simulink model "Project_3"  (R2020a)
settings: Solver=VariableStepAuto  StartTime=0.0  StopTime=10.0  RelTol=1e-3
settings Model: Creator=hp  LastModifiedBy=hp

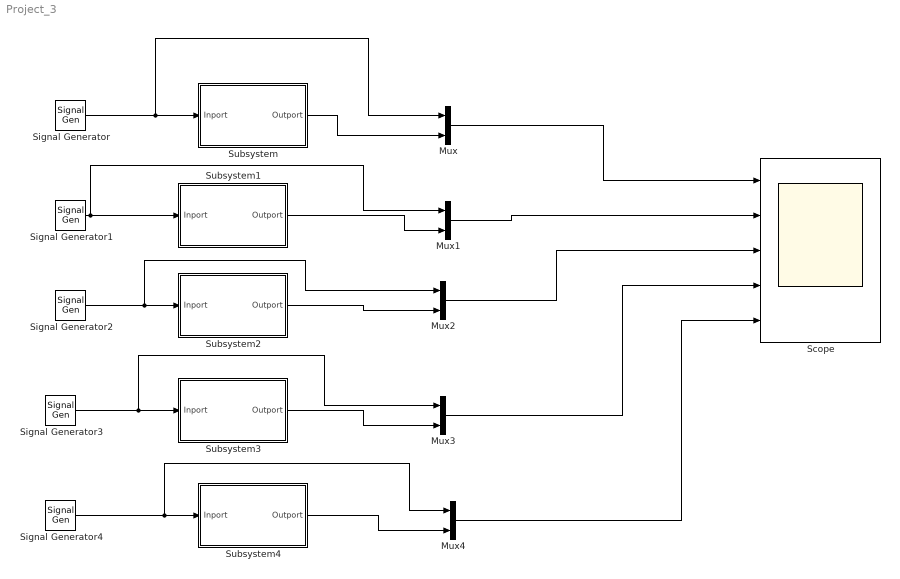
== system Project_3 ==
  Mux{,1..4} (5 alike) : Mux  Inputs=2
  Scope : Scope  NumInputPorts=5
  Signal Generator : SignalGenerator  Frequency=100
  Signal Generator1 : SignalGenerator  Frequency=200  Units=rad/sec
  Signal Generator2 : SignalGenerator  Frequency=500
  Signal Generator3 : SignalGenerator  Frequency=700
  Signal Generator4 : SignalGenerator  Frequency=1000
  Subsystem : Subsystem
  Subsystem1 : Subsystem
  Subsystem2 : Subsystem
  Subsystem3 : Subsystem
  Subsystem4 : Subsystem
  wires:
  Signal Generator4/1 -> Mux4/1, Subsystem4/1(Inport)
  Signal Generator3/1 -> Mux3/1, Subsystem3/1(Inport)
  Signal Generator2/1 -> Mux2/1, Subsystem2/1(Inport)
  Signal Generator/1 -> Mux/1, Subsystem/1(Inport)
  Subsystem/1(Outport) -> Mux/2
  Signal Generator1/1 -> Mux1/1, Subsystem1/1(Inport)
  Subsystem1/1(Outport) -> Mux1/2
  Subsystem2/1(Outport) -> Mux2/2
  Subsystem3/1(Outport) -> Mux3/2
  Subsystem4/1(Outport) -> Mux4/2
  Mux/1 -> Scope/1
  Mux1/1 -> Scope/2
  Mux2/1 -> Scope/3
  Mux3/1 -> Scope/4
  Mux4/1 -> Scope/5

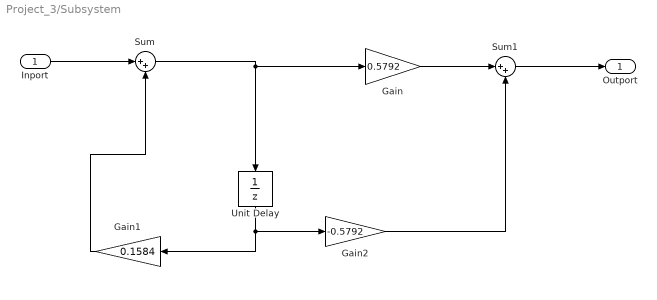
== system Project_3/Subsystem ==
  Inport : Inport
  Gain : Gain  Gain=0.5792
  Gain1 : Gain  Gain=0.1584
  Gain2 : Gain  Gain=-0.5792
  Sum : Sum  Inputs=|++
  Sum1 : Sum  Inputs=|++
  Unit Delay : UnitDelay  SampleTime=-1  HasFrameUpgradeWarning=on
  Outport : Outport
  wires:
  Gain/1 -> Sum1/1
  Gain1/1 -> Sum/2
  Unit Delay/1 -> Gain1/1, Gain2/1
  Gain2/1 -> Sum1/2
  Inport/1 -> Sum/1
  Sum1/1 -> Outport/1
  Sum/1 -> Unit Delay/1, Gain/1

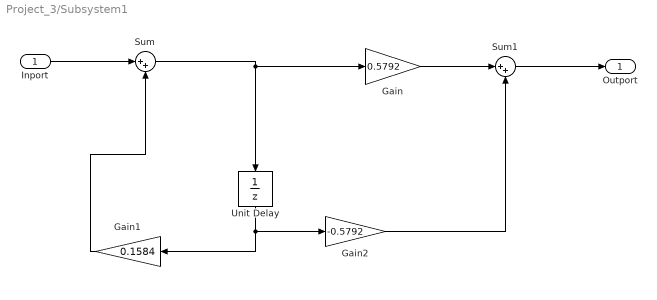
== system Project_3/Subsystem1 ==
  Inport : Inport
  Gain : Gain  Gain=0.5792
  Gain1 : Gain  Gain=0.1584
  Gain2 : Gain  Gain=-0.5792
  Sum : Sum  Inputs=|++
  Sum1 : Sum  Inputs=|++
  Unit Delay : UnitDelay  SampleTime=-1  HasFrameUpgradeWarning=on
  Outport : Outport
  wires:
  Gain/1 -> Sum1/1
  Gain1/1 -> Sum/2
  Unit Delay/1 -> Gain1/1, Gain2/1
  Gain2/1 -> Sum1/2
  Inport/1 -> Sum/1
  Sum1/1 -> Outport/1
  Sum/1 -> Unit Delay/1, Gain/1

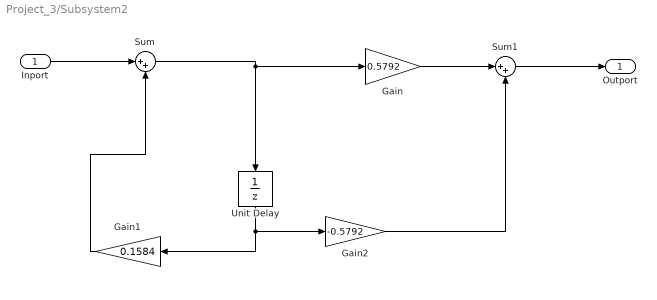
== system Project_3/Subsystem2 ==
  Inport : Inport
  Gain : Gain  Gain=0.5792
  Gain1 : Gain  Gain=0.1584
  Gain2 : Gain  Gain=-0.5792
  Sum : Sum  Inputs=|++
  Sum1 : Sum  Inputs=|++
  Unit Delay : UnitDelay  SampleTime=-1  HasFrameUpgradeWarning=on
  Outport : Outport
  wires:
  Gain/1 -> Sum1/1
  Gain1/1 -> Sum/2
  Unit Delay/1 -> Gain1/1, Gain2/1
  Gain2/1 -> Sum1/2
  Inport/1 -> Sum/1
  Sum1/1 -> Outport/1
  Sum/1 -> Unit Delay/1, Gain/1

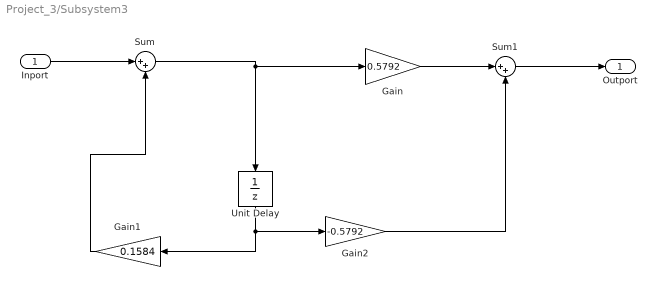
== system Project_3/Subsystem3 ==
  Inport : Inport
  Gain : Gain  Gain=0.5792
  Gain1 : Gain  Gain=0.1584
  Gain2 : Gain  Gain=-0.5792
  Sum : Sum  Inputs=|++
  Sum1 : Sum  Inputs=|++
  Unit Delay : UnitDelay  SampleTime=-1  HasFrameUpgradeWarning=on
  Outport : Outport
  wires:
  Gain/1 -> Sum1/1
  Gain1/1 -> Sum/2
  Unit Delay/1 -> Gain1/1, Gain2/1
  Gain2/1 -> Sum1/2
  Inport/1 -> Sum/1
  Sum1/1 -> Outport/1
  Sum/1 -> Unit Delay/1, Gain/1

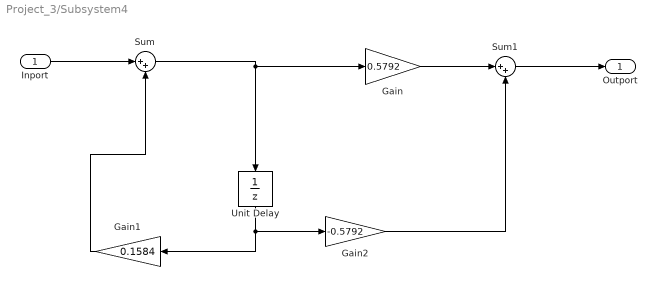
== system Project_3/Subsystem4 ==
  Inport : Inport
  Gain : Gain  Gain=0.5792
  Gain1 : Gain  Gain=0.1584
  Gain2 : Gain  Gain=-0.5792
  Sum : Sum  Inputs=|++
  Sum1 : Sum  Inputs=|++
  Unit Delay : UnitDelay  SampleTime=-1  HasFrameUpgradeWarning=on
  Outport : Outport
  wires:
  Gain/1 -> Sum1/1
  Gain1/1 -> Sum/2
  Unit Delay/1 -> Gain1/1, Gain2/1
  Gain2/1 -> Sum1/2
  Inport/1 -> Sum/1
  Sum1/1 -> Outport/1
  Sum/1 -> Unit Delay/1, Gain/1
